simulink library "Triped_utilities"  (R2020a)
settings: Solver=VariableStepAuto  StartTime=0.0  StopTime=10.0  RelTol=1e-3
values from neighbouring files (symbols this model uses):
  s = 1/(2*r)    [Weg0.m]
undefined symbols (not defined in the file or in its folder): X, Y, Z
libraries: sm_lib x8, powerlib_meascontrol x3, nesl_utility x3
settings Model: Creator=jan-b  LastModifiedBy=jan-b

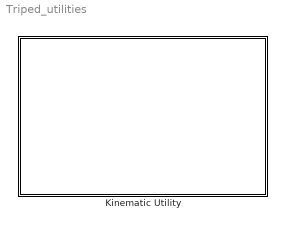
== system Triped_utilities ==
  Kinematic Utility : Subsystem

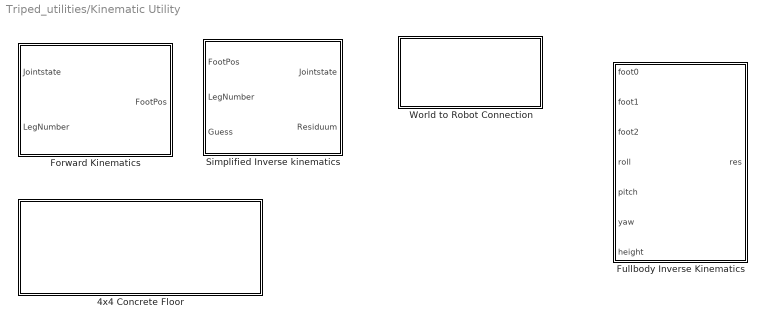
== system Triped_utilities/Kinematic Utility ==
  4x4 Concrete Floor : Subsystem
  Forward Kinematics : MATLAB Function  TreatAsAtomicUnit=on
  Fullbody Inverse Kinematics : MATLAB Function  TreatAsAtomicUnit=on
  Simplified Inverse kinematics : MATLAB Function  TreatAsAtomicUnit=on
  World to Robot Connection : Subsystem  Variant=on  VariantControlMode=Label  LabelModeActiveChoice=Choice_2

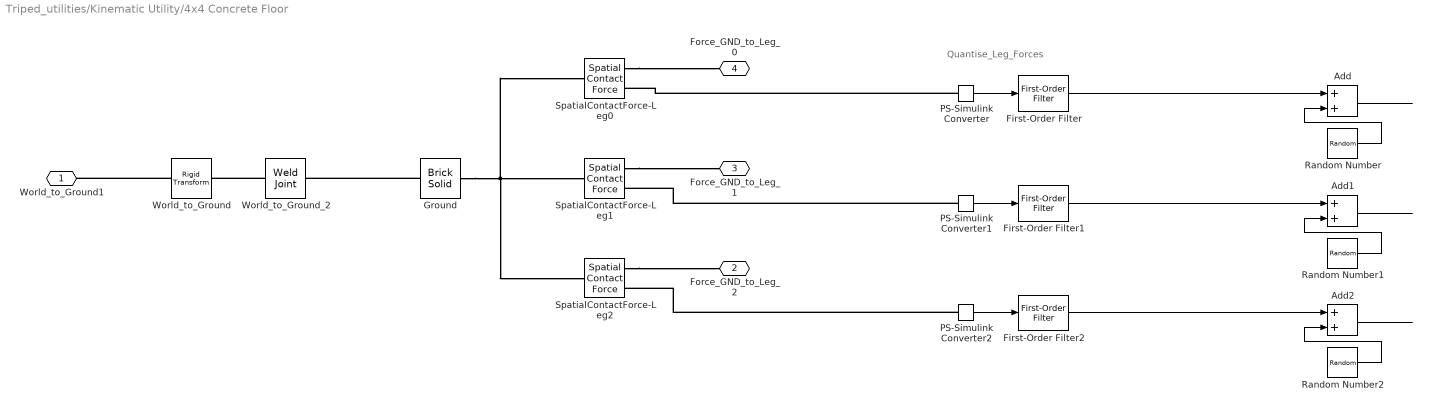
== system Triped_utilities/Kinematic Utility/4x4 Concrete Floor ==
  note: Quantise_Leg_Forces
  Add : Sum
  Add1 : Sum
  Add2 : Sum
  First-Order Filter : powerlib_meascontrol/Filters/First-Order Filter  FilterType=Lowpass  Tc=1/10  Ts=0  Initialize=on  Vac_Init=[0, 0, 60]  Vdc_Init=0  PlotResponse=off  FreqRange="[0,  200,  1]"
  First-Order Filter1 : powerlib_meascontrol/Filters/First-Order Filter  FilterType=Lowpass  Tc=1/10  Ts=0  Initialize=on  Vac_Init=[0, 0, 60]  Vdc_Init=0  PlotResponse=off  FreqRange="[0,  200,  1]"
  First-Order Filter2 : powerlib_meascontrol/Filters/First-Order Filter  FilterType=Lowpass  Tc=1/10  Ts=0  Initialize=on  Vac_Init=[0, 0, 60]  Vdc_Init=0  PlotResponse=off  FreqRange="[0,  200,  1]"
  Ground : sm_lib/Body Elements/Brick Solid  GraphicAmbientColor=[0.15 0.15 0.15 1.0]  BasedOnType=Density  BrickDimensions=[4 4 0.1]  BrickDimensionUnits=m  CenterOfMass=[0 0 0]  CenterOfMassUnits=m  GraphicDiffuseColor=[0.4 0.2 0.0]  Density=1000  DensityUnits=kg/m^3  DoExposeReferenceFrame=on  GraphicEmissiveColor=[0.0 0.0 0.0 1.0]  ExportEntireGeometry=on  SerializedFrames=<Frames/>  MarkerShape=Sphere  MarkerSize=10  GraphicType=FromGeometry  InertiaType=CalculateFromGeometry  Mass=1  MassUnits=kg  MomentsOfInertia=[1 1 1]  MomentsOfInertiaUnits=kg*m^2  GraphicOpacity=0.8  ProductsOfInertia=[0 0 0]  ProductsOfInertiaUnits=kg*m^2  GraphicShininess=75  GraphicSpecularColor=[0.5 0.5 0.5 1.0]  GraphicVisPropType=SimpleVisualProperties
  PS-Simulink Converter : nesl_utility/PS-Simulink Converter  PhysicalDomain=network_engine_domain  SubClassName=ps_output  LeftPortType=input  RightPortType=output  PseudoPeriodic=off  Frequencies=[]  Unit=inherit  AffineConversion=off
  PS-Simulink Converter1 : nesl_utility/PS-Simulink Converter  PhysicalDomain=network_engine_domain  SubClassName=ps_output  LeftPortType=input  RightPortType=output  PseudoPeriodic=off  Frequencies=[]  Unit=inherit  AffineConversion=off
  PS-Simulink Converter2 : nesl_utility/PS-Simulink Converter  PhysicalDomain=network_engine_domain  SubClassName=ps_output  LeftPortType=input  RightPortType=output  PseudoPeriodic=off  Frequencies=[]  Unit=inherit  AffineConversion=off
  Random Number : RandomNumber  Mean=1  Variance=0.002^2 /3
  Random Number1 : RandomNumber  Mean=1  Variance=0.002^2 /3
  Random Number2 : RandomNumber  Mean=1  Variance=0.002^2 /3
  SpatialContactForce-Leg0 : sm_lib/Forces and Torques/Spatial Contact Force  CoefficientOfDynamicFriction=0.8  CoefficientOfStaticFriction=1  NormalDamping=1e4  NormalDampingUnits=N/(m/s)  NormalStiffness=1e6  NormalStiffnessUnits=N/m  FrictionalCriticalVelocity=1e-3  FrictionalCriticalVelocityUnits=m/s  ZeroCrossDetectContactStartAndEnd=on  SenseFrictionalForceMagnitude=off  SenseNormalForceMagnitude=on  SenseSeparationDistance=off  NormalTransitionRegionWidth=1e-4  NormalTransitionRegionWidthUnits=m  FrictionType=SmoothStickSlip
  SpatialContactForce-Leg1 : sm_lib/Forces and Torques/Spatial Contact Force  CoefficientOfDynamicFriction=0.8  CoefficientOfStaticFriction=1  NormalDamping=1e4  NormalDampingUnits=N/(m/s)  NormalStiffness=1e6  NormalStiffnessUnits=N/m  FrictionalCriticalVelocity=1e-3  FrictionalCriticalVelocityUnits=m/s  ZeroCrossDetectContactStartAndEnd=on  SenseFrictionalForceMagnitude=off  SenseNormalForceMagnitude=on  SenseSeparationDistance=off  NormalTransitionRegionWidth=1e-4  NormalTransitionRegionWidthUnits=m  FrictionType=SmoothStickSlip
  SpatialContactForce-Leg2 : sm_lib/Forces and Torques/Spatial Contact Force  CoefficientOfDynamicFriction=0.8  CoefficientOfStaticFriction=1  NormalDamping=1e4  NormalDampingUnits=N/(m/s)  NormalStiffness=1e6  NormalStiffnessUnits=N/m  FrictionalCriticalVelocity=1e-3  FrictionalCriticalVelocityUnits=m/s  ZeroCrossDetectContactStartAndEnd=on  SenseFrictionalForceMagnitude=off  SenseNormalForceMagnitude=on  SenseSeparationDistance=off  NormalTransitionRegionWidth=1e-4  NormalTransitionRegionWidthUnits=m  FrictionType=SmoothStickSlip
  World_to_Ground : sm_lib/Frames and Transforms/Rigid Transform  TranslationMethod=Cartesian  TranslationStandardOffset=0  TranslationLengthUnit=m  TranslationStandardAxis=+Z  TranslationCartesianOffset=[0 0 -0.5]  TranslationROffset=0  TranslationROffsetUnits=m  TranslationZOffset=0  TranslationZOffsetUnits=m  TranslationThetaOffset=0  TranslationThetaOffsetUnits=deg  RotationMethod=None  RotationAngleUnits=deg  RotationStandardAxis=+Z  RotationAngle=0.0  RotationArbitraryAxis=[0 0 1]  FollAlignAxisA=+X  BaseAlignAxisA=+Y  FollAlignAxisB=+Y  BaseAlignAxisB=+Z  RotationSequenceAxes=FollowerAxes  RotationSequence=XYX  RotationSequenceAngles=[0 0 0]  RotationSequenceAnglesUnits=deg  RotationMatrix=[1 0 0; 0 1 0; 0 0 1]
  World_to_Ground_2 : sm_lib/Joints/Weld Joint  JointMode=Normal  SenseConstraintForce=off  SenseConstraintForceX=off  SenseConstraintForceY=off  SenseConstraintForceZ=off  SenseConstraintTorque=off  SenseConstraintTorqueX=off  SenseConstraintTorqueY=off  SenseConstraintTorqueZ=off  SenseTotalForce=off  SenseTotalForceX=off  SenseTotalForceY=off  SenseTotalForceZ=off  SenseTotalTorque=off  SenseTotalTorqueX=off  SenseTotalTorqueY=off  SenseTotalTorqueZ=off  CompositeWrenchDir=FollowerOnBase  CompositeWrenchFrame=BaseFrame
  World_to_Ground1 : PMIOPort  Side=Left
  Force_GND_to_Leg_2 : PMIOPort  Port=2  Side=Right
  Force_GND_to_Leg_1 : PMIOPort  Port=3  Side=Right
  Force_GND_to_Leg_0 : PMIOPort  Port=4  Side=Right
  wires:
  First-Order Filter2/1 -> Add2/1
  First-Order Filter1/1 -> Add1/1
  First-Order Filter/1 -> Add/1
  Add2/1 -> ?
  PS-Simulink Converter2/1 -> First-Order Filter2/1
  Random Number2/1 -> Add2/2
  Add1/1 -> ?
  PS-Simulink Converter1/1 -> First-Order Filter1/1
  Random Number1/1 -> Add1/2
  PS-Simulink Converter/1 -> First-Order Filter/1
  Random Number/1 -> Add/2
  Add/1 -> ?
  connections:
  Ground/RConn1 -- World_to_Ground_2/RConn1
  Ground/LConn1 -- SpatialContactForce-Leg0/LConn1 -- SpatialContactForce-Leg1/LConn1 -- SpatialContactForce-Leg2/LConn1
  SpatialContactForce-Leg1/RConn1 -- Force_GND_to_Leg_1/RConn1
  World_to_Ground/LConn1 -- World_to_Ground1/RConn1
  SpatialContactForce-Leg2/RConn1 -- Force_GND_to_Leg_2/RConn1
  SpatialContactForce-Leg0/RConn1 -- Force_GND_to_Leg_0/RConn1
  World_to_Ground_2/LConn1 -- World_to_Ground/RConn1
  PS-Simulink Converter1/LConn1 -- SpatialContactForce-Leg1/RConn2
  PS-Simulink Converter2/LConn1 -- SpatialContactForce-Leg2/RConn2
  PS-Simulink Converter/LConn1 -- SpatialContactForce-Leg0/RConn2

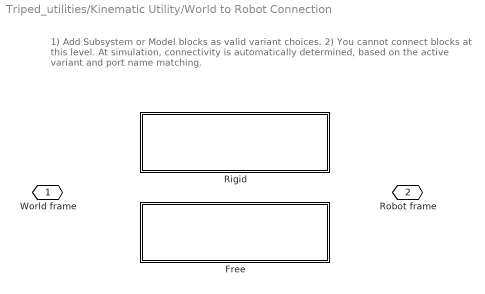
== system Triped_utilities/Kinematic Utility/World to Robot Connection ==
  note: 1) Add Subsystem or Model blocks as valid variant choices.
      | 2) You cannot connect blocks at this level. At simulation, connectivity is automatically
      | determined, based on the active variant and port name matching.
  Free : Subsystem  VariantControl=Choice_2
  Rigid : Subsystem  VariantControl=(default)
  World frame : PMIOPort  Side=Left
  Robot frame : PMIOPort  Port=2  Side=Right

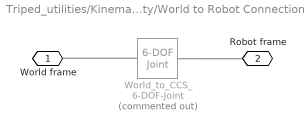
== system Triped_utilities/Kinematic Utility/World to Robot Connection/Free ==
  World_to_CCS_6-DOF-Joint : sm_lib/Joints/6-DOF Joint  Commented=on  JointMode=Normal  SenseConstraintForce=off  SenseConstraintForceX=off  SenseConstraintForceY=off  SenseConstraintForceZ=off  SenseConstraintTorque=off  SenseConstraintTorqueX=off  SenseConstraintTorqueY=off  SenseConstraintTorqueZ=off  SenseTotalForce=off  SenseTotalForceX=off  SenseTotalForceY=off  SenseTotalForceZ=off  SenseTotalTorque=off  SenseTotalTorqueX=off  SenseTotalTorqueY=off  SenseTotalTorqueZ=off  CompositeWrenchDir=FollowerOnBase  CompositeWrenchFrame=BaseFrame  PxEquilibriumPosition=0  PxEquilibriumPositionUnits=m  PxSpringStiffness=0  PxSpringStiffnessUnits=N/m  PxDampingCoefficient=0  PxDampingCoefficientUnits=N/(m/s)  PxTorqueActuationMode=NoTorque  PxMotionActuationMode=ComputedMotion  PxSensePosition=off  PxSenseVelocity=off  PxSenseAcceleration=off  PxSenseTorqueForce=off  PxSenseLowerLimitTorqueForce=off  PxSenseUpperLimitTorqueForce=off  PxLowerLimitSpecify=off  PxLowerLimitBound=-1  PxLowerLimitBoundUnits=m  PxLowerLimitStiffness=1e6  PxLowerLimitStiffnessUnits=N/m  PxLowerLimitDamping=1e3  PxLowerLimitDampingUnits=N/(m/s)  PxLowerLimitTransitionRegionWidth=1e-4  PxLowerLimitTransitionRegionWidthUnits=m  PxUpperLimitSpecify=off  PxUpperLimitBound=1  PxUpperLimitBoundUnits=m  PxUpperLimitStiffness=1e6  PxUpperLimitStiffnessUnits=N/m  PxUpperLimitDamping=1e3  PxUpperLimitDampingUnits=N/(m/s)  PxUpperLimitTransitionRegionWidth=1e-4  PxUpperLimitTransitionRegionWidthUnits=m  PxPositionTargetSpecify=off  PxPositionTargetPriority=High  PxPositionTargetValue=0  PxPositionTargetValueUnits=m  PxVelocityTargetSpecify=off  PxVelocityTargetPriority=High  PxVelocityTargetValue=0  PxVelocityTargetValueUnits=m/s  PyEquilibriumPosition=0  PyEquilibriumPositionUnits=m  PySpringStiffness=0  PySpringStiffnessUnits=N/m  PyDampingCoefficient=0  PyDampingCoefficientUnits=N/(m/s)  PyTorqueActuationMode=NoTorque  PyMotionActuationMode=ComputedMotion  PySensePosition=off  PySenseVelocity=off  PySenseAcceleration=off  PySenseTorqueForce=off  PySenseLowerLimitTorqueForce=off  PySenseUpperLimitTorqueForce=off  PyLowerLimitSpecify=off  PyLowerLimitBound=-1  PyLowerLimitBoundUnits=m  PyLowerLimitStiffness=1e6  PyLowerLimitStiffnessUnits=N/m  PyLowerLimitDamping=1e3  PyLowerLimitDampingUnits=N/(m/s)  PyLowerLimitTransitionRegionWidth=1e-4  PyLowerLimitTransitionRegionWidthUnits=m  PyUpperLimitSpecify=off  PyUpperLimitBound=1  PyUpperLimitBoundUnits=m  PyUpperLimitStiffness=1e6  PyUpperLimitStiffnessUnits=N/m  PyUpperLimitDamping=1e3  PyUpperLimitDampingUnits=N/(m/s)  PyUpperLimitTransitionRegionWidth=1e-4  PyUpperLimitTransitionRegionWidthUnits=m  PyPositionTargetSpecify=off  PyPositionTargetPriority=High  PyPositionTargetValue=0  PyPositionTargetValueUnits=m  PyVelocityTargetSpecify=off  PyVelocityTargetPriority=High  PyVelocityTargetValue=0  PyVelocityTargetValueUnits=m/s  PzEquilibriumPosition=0  PzEquilibriumPositionUnits=m  PzSpringStiffness=0  PzSpringStiffnessUnits=N/m  PzDampingCoefficient=0  PzDampingCoefficientUnits=N/(m/s)  PzTorqueActuationMode=NoTorque  PzMotionActuationMode=ComputedMotion  PzSensePosition=off  PzSenseVelocity=off  PzSenseAcceleration=off  PzSenseTorqueForce=off  PzSenseLowerLimitTorqueForce=off  PzSenseUpperLimitTorqueForce=off  PzLowerLimitSpecify=off  PzLowerLimitBound=-1  PzLowerLimitBoundUnits=m  PzLowerLimitStiffness=1e6  PzLowerLimitStiffnessUnits=N/m  PzLowerLimitDamping=1e3  PzLowerLimitDampingUnits=N/(m/s)  PzLowerLimitTransitionRegionWidth=1e-4  PzLowerLimitTransitionRegionWidthUnits=m  PzUpperLimitSpecify=off  PzUpperLimitBound=1  PzUpperLimitBoundUnits=m  PzUpperLimitStiffness=1e6  PzUpperLimitStiffnessUnits=N/m  PzUpperLimitDamping=1e3  PzUpperLimitDampingUnits=N/(m/s)  PzUpperLimitTransitionRegionWidth=1e-4  PzUpperLimitTransitionRegionWidthUnits=m  PzPositionTargetSpecify=off  PzPositionTargetPriority=High  PzPositionTargetValue=0  PzPositionTargetValueUnits=m  PzVelocityTargetSpecify=off  PzVelocityTargetPriority=High  PzVelocityTargetValue=0  PzVelocityTargetValueUnits=m/s  SphDefPosRotationMethod=None  SphDefPosRotationAngleUnits=deg  SphDefPosRotationStandardAxis=+Z  SphDefPosRotationAngle=0.0  SphDefPosRotationArbitraryAxis=[0 0 1]  SphDefPosFollAlignAxisA=+X  SphDefPosBaseAlignAxisA=+Y  SphDefPosFollAlignAxisB=+Y  SphDefPosBaseAlignAxisB=+Z  SphDefPosRotationSequenceAxes=FollowerAxes  SphDefPosRotationSequence=XYX  SphDefPosRotationSequenceAngles=[0 0 0]  SphDefPosRotationSequenceAnglesUnits=deg  SphDefPosRotationMatrix=[1 0 0; 0 1 0; 0 0 1]  SphEqPosRotationMethod=None  SphEqPosRotationAngleUnits=deg  SphEqPosRotationStandardAxis=+Z  SphEqPosRotationAngle=0.0  SphEqPosRotationArbitraryAxis=[0 0 1]  SphEqPosFollAlignAxisA=+X  SphEqPosBaseAlignAxisA=+Y  SphEqPosFollAlignAxisB=+Y  SphEqPosBaseAlignAxisB=+Z  SphEqPosRotationSequenceAxes=FollowerAxes  SphEqPosRotationSequence=XYX  SphEqPosRotationSequenceAngles=[0 0 0]  SphEqPosRotationSequenceAnglesUnits=deg  SphEqPosRotationMatrix=[1 0 0; 0 1 0; 0 0 1]  SphSpringStiffness=0  SphSpringStiffnessUnits=N*m/deg  SphDampingCoefficient=0  SphDampingCoefficientUnits=N*m/(deg/s)  SphActuateTorqueX=off  SphActuateTorqueY=off  SphActuateTorqueZ=off  SphActuateTorque=off  SphTorqueActuationMode=NoTorque  SphMotionActuationMode=ComputedMotion  SphActuationFrame=BaseFrame  SphSensePosition=off  SphSenseVelocityX=off  SphSenseVelocityY=off  SphSenseVelocityZ=off  SphSenseVelocity=off  SphSenseAccelerationX=off  SphSenseAccelerationY=off  SphSenseAccelerationZ=off  SphSenseAcceleration=off  SphSenseTorqueX=off  SphSenseTorqueY=off  SphSenseTorqueZ=off  SphSenseTorqueForce=off  SphSenseLowerLimitTorqueMag=off  SphSenseUpperLimitTorqueMag=off  SphSensingFrame=BaseFrame  SphLowerLimitSpecify=off  SphLowerLimitBound=15  SphLowerLimitBoundUnits=deg  SphLowerLimitStiffness=1e4  SphLowerLimitStiffnessUnits=N*m/deg  SphLowerLimitDamping=10  SphLowerLimitDampingUnits=N*m/(deg/s)  SphLowerLimitTransitionRegionWidth=0.1  SphLowerLimitTransitionRegionWidthUnits=deg  SphUpperLimitSpecify=off  SphUpperLimitBound=45  SphUpperLimitBoundUnits=deg  SphUpperLimitStiffness=1e4  SphUpperLimitStiffnessUnits=N*m/deg  SphUpperLimitDamping=10  SphUpperLimitDampingUnits=N*m/(deg/s)  SphUpperLimitTransitionRegionWidth=0.1  SphUpperLimitTransitionRegionWidthUnits=deg  SphPositionTargetRotationMethod=None  SphPositionTargetRotationAngleUnits=deg  SphPositionTargetRotationStandardAxis=+Z  SphPositionTargetRotationAngle=0.0  SphPositionTargetRotationArbitraryAxis=[0 0 1]  SphPositionTargetFollAlignAxisA=+X  SphPositionTargetBaseAlignAxisA=+Y  SphPositionTargetFollAlignAxisB=+Y  SphPositionTargetBaseAlignAxisB=+Z  SphPositionTargetRotationSequenceAxes=FollowerAxes  SphPositionTargetRotationSequence=XYX  SphPositionTargetRotationSequenceAngles=[0 0 0]  SphPositionTargetRotationSequenceAnglesUnits=deg  SphPositionTargetRotationMatrix=[1 0 0; 0 1 0; 0 0 1]  SphPositionTargetSpecify=off  SphPositionTargetPriority=High  SphVelocityTargetValue=[0 0 0]  SphVelocityTargetValueUnits=deg/s  SphVelocityTargetSpecify=off  SphVelocityTargetPriority=High  SphVelocityTargetInFollowerFrame=on
  World frame : PMIOPort  Side=Left
  Robot frame : PMIOPort  Port=2  Side=Right
  connections:
  World_to_CCS_6-DOF-Joint/RConn1 -- Robot frame/RConn1
  World_to_CCS_6-DOF-Joint/LConn1 -- World frame/RConn1

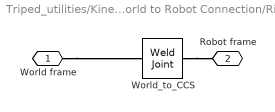
== system Triped_utilities/Kinematic Utility/World to Robot Connection/Rigid ==
  World_to_CCS : sm_lib/Joints/Weld Joint  JointMode=Normal  SenseConstraintForce=off  SenseConstraintForceX=off  SenseConstraintForceY=off  SenseConstraintForceZ=off  SenseConstraintTorque=off  SenseConstraintTorqueX=off  SenseConstraintTorqueY=off  SenseConstraintTorqueZ=off  SenseTotalForce=off  SenseTotalForceX=off  SenseTotalForceY=off  SenseTotalForceZ=off  SenseTotalTorque=off  SenseTotalTorqueX=off  SenseTotalTorqueY=off  SenseTotalTorqueZ=off  CompositeWrenchDir=FollowerOnBase  CompositeWrenchFrame=BaseFrame
  World frame : PMIOPort  Side=Left
  Robot frame : PMIOPort  Port=2  Side=Right
  connections:
  World_to_CCS/RConn1 -- Robot frame/RConn1
  World frame/RConn1 -- World_to_CCS/LConn1

== matlab function Triped_utilities/Kinematic Utility/Simplified Inverse kinematics ==
  data: Jointstate output; FootPos input; LegNumber input; Guess input; Residuum output
function [Jointstate,Residuum]= fcn(FootPos,LegNumber, Guess)



% easy adapt to legs 1 & 2: change base coordinate system from ccs, to
% rotated ccs.
x=FootPos(1);
y=FootPos(2);
z=FootPos(3);
[newx,newy,newz] = transformCoordinateSystem(x,y,z,LegNumber);

% calculate target Matrix from input cordinates
%reduced task space to x,y,z, ignore roll, pitch, yaw
[targetM] = convertCoordinatesToMatrix(newx,newy,newz);

%convert euer angles from data to quaternion
guess = convertDataToGuess(Guess);

[extend, a0,b0,c0,d0, Residuum] = inverseKinematics(targetM,guess);
eulerXYZ = quat2eul([a0,b0,c0,d0],'XYZ');
Rx = eulerXYZ(1);
Ry = eulerXYZ(2);
Rz = eulerXYZ(3);
Jointstate=[ extend, Rx,Ry,Rz];
end

function [newx,newy,newz] = transformCoordinateSystem(oldx,oldy,oldz,legNr)
% this function translates the x,y,z coordinates from the CCS into
% coordinates from a cooridnate system, which is like the ccs but rotated
% ,such that its x axis points towards the leg. This makes the inverse
% kinematics for the leg 1 & 2 easier.

angle = legNr * 120 * pi/180;

newCoord = [cos(angle), -sin(angle), 0, 0; sin(angle), cos(angle), 0, 0; 0, 0, 1, 0; 0, 0, 0, 1]* [oldx;oldy;oldz;1];
newx = newCoord(1);
newy = newCoord(2);
newz = newCoord(3);

end

function [transfM] = convertCoordinatesToMatrix(x,y,z)
% roll = rotX, pitch  = rotY, yaw = rotZ 

%first translate frame by [x,y,z]
transfM = homogenTranslationMat(x,y,z);

%then rotate using the roll-pitch-yaw convention
%transfM2 = eul2rotm([roll,pitch,yaw],'XYZ');
%transfM2 =  [transfM2,[0;0;0];[0,0,0,1]];

%transfM = transfM1 * transfM2;

end

function [guess] = convertDataToGuess(data)
    qXYZ = eul2quat([data(1),data(2),data(3)],'XYZ');
    guess = [qXYZ,data(4)];
    
end

function [theta0,a0,b0,c0,d0,fvalWay0] = inverseKinematics(A,guess)
% maps a homogene transformation matrix, which describes a position and
% orientation from the fcs relative to the ccs, to the joint space
% variables
% tldr: Matrix A -> values for MCS00/01/02

options = optimoptions(@fmincon,'OptimalityTolerance',10^-10,'StepTolerance',10^-10,'display','off','Algorithm','sqp'); % some options for more precise solution

% find out transformation matrix for way0 & LL such that the error to A is
% minimal
% guessTheta0 = 0 * pi / 180;
%guessTheta0 = sim_theta0;
% arbitrary quess values. should be somewhat in the right area.
%guessVals = [0.9961, -0.0000, -0.0893, 0.0000, guessTheta0]; % [a0,b0,c0,d0,theta0]
guessVals = guess;

% disp('Minimizing way 0 + LL');
%[OptVals,fval,~,output] = fminunc(@closingWay0toTarget,guessVals,options)
clW0toTarget = @(guessVals)closingWay0toTarget(guessVals,A);
[OptVals,fvalWay0,~,~] = fmincon(clW0toTarget,guessVals,[],[],[],[],[],[],@constrainsWay0,options);

% get values from way0
a0 = OptVals(1);
b0 = OptVals(2);
c0 = OptVals(3);
d0 = OptVals(4);
theta0 = OptVals(5);

end


function [error] = closingWay0toTarget(GUESSEDVALS,MatA)
% this function returns the error between the joint values of the kinematic
% way 0 with added LegLinear ( CCS -> LCS0 --> FCS) and the joint values of
% the target matrix MatA


a0 = GUESSEDVALS(1);
b0 = GUESSEDVALS(2);
c0 = GUESSEDVALS(3);
d0 = GUESSEDVALS(4);
theta0 = GUESSEDVALS(5);

way0m = Weg0(a0,b0,c0,d0);
way0LLm = AddLegLinear(way0m,theta0);
[a,b,c,d, x,y,z] = getValuesfromHomogenMatrix(way0LLm);
[Aa,Ab,Ac,Ad, Ax,Ay,Az] = getValuesfromHomogenMatrix(MatA);

error = sum(([a,b,c,d, x,y,z] - [Aa,Ab,Ac,Ad, Ax,Ay,Az]).^2) + 1000*(a^2+b^2+c^2+d^2 -1)^2; % error of the transform to A. we want to minimze this
end


function [c,ceq]= constrainsWay0(x)
% make sure that solver fmincon, solves with constraint : ||quat0|| == 1
%input: x = [a0,b0,c0,d0,theta0]. with a to d parameters of quat0
c = []; % condition for ... <= 0
ceq = x(1)^2+x(2)^2+x(3)^2+x(4)^2 - 1; % condition for ||quat0|| == 1    
end

function [Weg0Mat] = Weg0(a0,b0,c0,d0)
A1 = homogenTranslationMat(0.265,0,0.014);
A2 = makeRotHomogen(quatRotM(a0,b0,c0,d0));
Weg0Mat = A1 * A2;
end

function [ALeg] = AddLegLinear(A,theta0)
% this functions adds transformations from the Point P; which is the
% Endpoint from Weg0,1,2; to the FKS at the LegLinear part.
%{
Inputs:
A: Transformationmatrix, which describes Transformation from HKS to P, Use
Weg0.m for that.
theta0: angle [radians] for joint at MKS00
%}

A1 = homogenTranslationMat(1.640, 0, -0.037); % transform P to P0 (center of LegLinear rotation)

theta0 = -1* theta0 * 0.07/(2*pi*1.5); % gear constraint: transfrom theta at MKS00 to theta around P0, gear ratio is 0.07/(2*pi*1.5) [circumferences of the gears MCS00 / LL]
startingvalue = -0 * pi/180;
theta0 = theta0 + startingvalue; %offset, depending on which position the Leg is for theta at MKS00 is 0
A2 = makeRotHomogen(quatRotM(cos(theta0/2),0,sin(theta0/2),0)); % rotate theta [radians] around y-axis of P0

A3 = homogenTranslationMat(-1.500,0,0); %transform from P0-joint to FKS

ALeg = A*A1*A2*A3;
end

function [res] = homogenTranslationMat(x,y,z)
    %this function forms a Translation about a vector x,y,z in a homogenous
    %transformation matrix res. 
    res = [1 0 0 x; 0 1 0 y; 0 0 1 z; 0 0 0 1];
end

function [res] = makeRotHomogen(R)
% this function fills a Rotationmatrix to make it a homogen transformation
% matrix
res = [R(1,1) R(1,2) R(1,3) 0; R(2,1) R(2,2) R(2,3) 0; R(3,1) R(3,2) R(3,3) 0; 0 0 0 1];
end

function [res] = quatRotM(a,b,c,d) %%Todo: use a,b,c,d as inputs
    % this function calculates the quaternion rotation matrix for given
    % vector (kx,ky,kz) and angle theta
    res = [1-2*(c^2+d^2) 2*(b*c-d*a) 2*(b*d + c*a); 2*(b*c + d*a) 1-2*(b^2+d^2) 2*(c*d - b*a); 2*(b*d-c*a) 2*(c*d+b*a) 1-2*(b^2+c^2) ];
end

function [a,b,c,d, x,y,z] = getValuesfromHomogenMatrix(A)
    % this function returns the Vector by which a homogenous
    % Transformationmatrix shifts a Point
    x = A(1,4);
    y = A(2,4);
    z = A(3,4);

    %as well as the Values of the Quaternion describing the rotation
    R = A(1:3,1:3); % get Rot mat from homogen Mat
    
    t = R(1,1)+R(2,2)+R(3,3);
    r = sqrt(1+t);
    s = 1/(2*r);
    a = 1/2 * r;
    b = (R(3,2)-R(2,3))*s;
    c = (R(1,3)-R(3,1))*s;
    d= (R(2,1)-R(1,2))*s;
    
end

== matlab function Triped_utilities/Kinematic Utility/Forward Kinematics ==
  data: Jointstate input; FootPos output; LegNumber input
function FootPos = fcn(Jointstate, LegNumber)
waym = Weg0(eul2quat(Jointstate(1:3).','XYZ'));
wayLLm = AddLegLinear(waym,Jointstate(4));
legstate = getPosfromHomogenMatrix(wayLLm);
leg_pos = transformCoordinateSystem(legstate(1),legstate(2),legstate(3),LegNumber);


FootPos = leg_pos;
end




function [new_pos] = transformCoordinateSystem(oldx,oldy,oldz,legNr)
% this function translates the x,y,z coordinates from the CCS into
% coordinates from a cooridnate system, which is like the ccs but rotated
% ,such that its x axis points towards the leg. This makes the inverse
% kinematics for the leg 1 & 2 easier.

angle = legNr * 120 * pi/180;

newCoord = [cos(angle), -sin(angle), 0, 0; sin(angle), cos(angle), 0, 0; 0, 0, 1, 0; 0, 0, 0, 1]* [oldx;oldy;oldz;1];
newx = newCoord(1);
newy = newCoord(2);
newz = newCoord(3);

new_pos=[newx;newy;newz];
end

function [Weg0Mat] = Weg0(quat)
a0=quat(1);
b0=quat(2);
c0=quat(3);
d0=quat(4)
A1 = homogenTranslationMat(0.265,0,0.014);
A2 = makeRotHomogen(quatRotM(a0,b0,c0,d0));
Weg0Mat = A1 * A2;
end



function [ALeg] = AddLegLinear(A,theta0)
% this functions adds transformations from the Point P; which is the
% Endpoint from Weg0,1,2; to the FKS at the LegLinear part.
%{
Inputs:
A: Transformationmatrix, which describes Transformation from HKS to P, Use
Weg0.m for that.
theta0: angle [radians] for joint at MKS00
%}

A1 = homogenTranslationMat(1.640, 0, -0.037); % transform P to P0 (center of LegLinear rotation)

theta0 = -1* theta0 * 0.07/(2*pi*1.5); % gear constraint: transfrom theta at MKS00 to theta around P0, gear ratio is 0.07/(2*pi*1.5) [circumferences of the gears MCS00 / LL]
startingvalue = -0 * pi/180;
theta0 = theta0 + startingvalue; %offset, depending on which position the Leg is for theta at MKS00 is 0
A2 = makeRotHomogen(quatRotM(cos(theta0/2),0,sin(theta0/2),0)); % rotate theta [radians] around y-axis of P0

A3 = homogenTranslationMat(-1.500,0,0); %transform from P0-joint to FKS

ALeg = A*A1*A2*A3;
end

function [res] = homogenTranslationMat(x,y,z)
    %this function forms a Translation about a vector x,y,z in a homogenous
    %transformation matrix res. 
    res = [1 0 0 x; 0 1 0 y; 0 0 1 z; 0 0 0 1];
end

function [res] = makeRotHomogen(R)
% this function fills a Rotationmatrix to make it a homogen transformation
% matrix
res = [R(1,1) R(1,2) R(1,3) 0; R(2,1) R(2,2) R(2,3) 0; R(3,1) R(3,2) R(3,3) 0; 0 0 0 1];
end

function [res] = quatRotM(a,b,c,d) %%Todo: use a,b,c,d as inputs
    % this function calculates the quaternion rotation matrix for given
    % vector (kx,ky,kz) and angle theta
    res = [1-2*(c^2+d^2) 2*(b*c-d*a) 2*(b*d + c*a); 2*(b*c + d*a) 1-2*(b^2+d^2) 2*(c*d - b*a); 2*(b*d-c*a) 2*(c*d+b*a) 1-2*(b^2+c^2) ];
end

function [a,b,c,d, x,y,z] = getValuesfromHomogenMatrix(A)
    % this function returns the Vector by which a homogenous
    % Transformationmatrix shifts a Point
    x = A(1,4);
    y = A(2,4);
    z = A(3,4);

    %as well as the Values of the Quaternion describing the rotation
    R = A(1:3,1:3); % get Rot mat from homogen Mat
    
    t = R(1,1)+R(2,2)+R(3,3);
    r = sqrt(1+t);
    s = 1/(2*r);
    a = 1/2 * r;
    b = (R(3,2)-R(2,3))*s;
    c = (R(1,3)-R(3,1))*s;
    d= (R(2,1)-R(1,2))*s;
end


function [pos] = getPosfromHomogenMatrix(A)
    % this function returns the Vector by which a homogenous
    % Transformationmatrix shifts a Point
    x = A(1,4);
    y = A(2,4);
    z = A(3,4);

    pos=[x,y,z]
end

== matlab function Triped_utilities/Kinematic Utility/Fullbody Inverse Kinematics ==
  data: foot0 input; res output; foot1 input; foot2 input; roll input; pitch input; yaw input; height input
function res  = fcn(foot0,foot1,foot2,roll,pitch,yaw,height)
floor_ccs_trafo=transform_to_floor(roll,pitch,yaw,height);

ccs_foot0=floor_ccs_trafo*makehomogenous(foot0);
ccs_foot1=floor_ccs_trafo*makehomogenous(foot1);
ccs_foot2=floor_ccs_trafo*makehomogenous(foot2);
res=[ccs_foot0(1:3);ccs_foot1(1:3);ccs_foot2(1:3)];
end


function [transfM] = transform_to_floor(roll,pitch,yaw,height)
%first translate frame by [x,y,z]
transfM1 = homogenTranslationMat(0,0,-height);
%then rotate using the roll-pitch-yaw convention
transfM2 = makeRotHomogen(eul2rotm([-roll,-pitch,-yaw],'XYZ'));
transfM = transfM1 * transfM2;
end

function [res] = makehomogenous(vector)
    res = [vector(1);vector(2);vector(3);1];
end

function [res] = homogenTranslationMat(x,y,z)
    %this function forms a Translation about a vector x,y,z in a homogenous
    %transformation matrix res. 
    res = [1 0 0 x; 0 1 0 y; 0 0 1 z; 0 0 0 1];
end

function [res] = makeRotHomogen(R)
% this function fills a Rotationmatrix to make it a homogen transformation
% matrix
res = [R(1,1) R(1,2) R(1,3) 0; R(2,1) R(2,2) R(2,3) 0; R(3,1) R(3,2) R(3,3) 0; 0 0 0 1];
end
